simulink model "retro_pid_rootlocus_freq"  (R2021a)
settings: Solver=VariableStepAuto  StartTime=0.0  StopTime=10.0  RelTol=1e-3
values from neighbouring files (symbols this model uses):
  b = 0.1    [controlloPID.m]    (also in modello_CA.m)
  g = 9.8    [controlloPID.m]    (also in modello2.m = 9.81; modello_CA.m = 9.81)
  i = 0.006    [controlloPID.m]    (also in modello_CA.m = 0.00030246)
  Ki = 1    [controlloPID.m]    (also in modello_CA.m = 177.3)
  Kp = 100    [controlloPID.m]    (also in modello_CA.m = 27.59)
  M = 0.5    [controlloPID.m]    (also in modello2.m = 0.04; modello_CA.m = 0.04)
  m = 0.2    [controlloPID.m]    (also in modello2.m = 0.06; modello_CA.m = 0.06)
undefined symbols (not defined in the file or in its folder): k
libraries: pid_lib x1
settings Model: Creator=olegg  LastModifiedBy=olegg

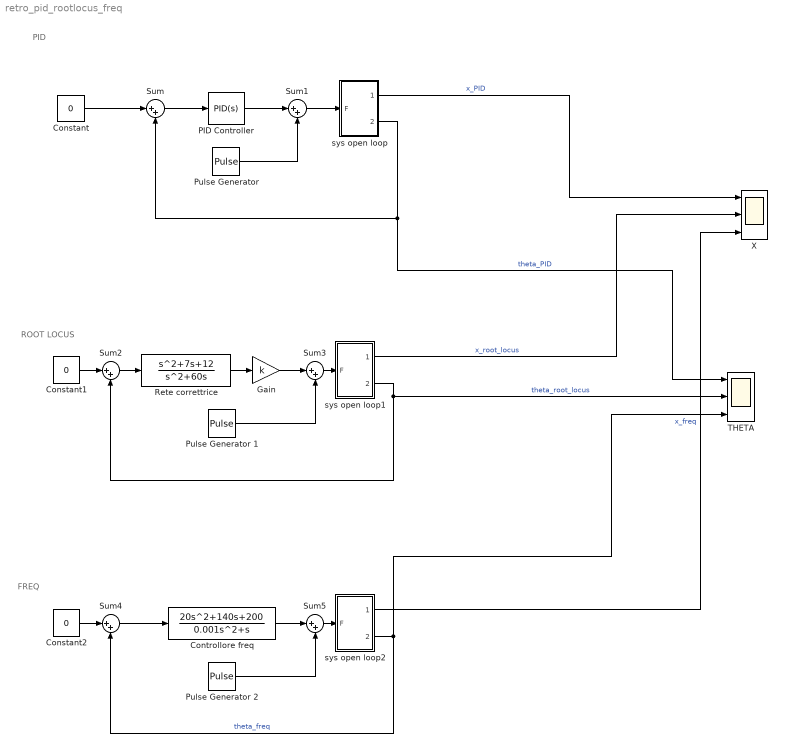
== system retro_pid_rootlocus_freq ==
  note: FREQ
  note: ROOT LOCUS
  note: PID
  Constant : Constant  Value=0
  Constant1 : Constant  Value=0
  Constant2 : Constant  Value=0
  Controllore freq : TransferFcn  Numerator=[20 140 200]  Denominator=[0.001 1 0]
  Gain : Gain  Gain=k
  PID Controller : pid_lib/PID Controller  Controller=PID  Form=Parallel  TimeDomain=Continuous-time  UseExternalTs=off  SampleTime=-1  IntegratorMethod=Forward Euler  FilterMethod=Forward Euler  ControllerParametersSource=internal  P=Kp  I=Ki  D=Kp  UseFilter=on  N=100  TunerSelectOption=Transfer Function Based (PID Tuner App)  InitialConditionSource=internal  InitialConditionForIntegrator=0  InitialConditionForFilter=0  DifferentiatorICPrevScaledInput=0  ExternalReset=none  TrackingMode=off  Kt=1  LimitOutput=off  SatLimitsSource=internal  UpperSaturationLimit=inf  LowerSaturationLimit=-inf  LinearizeAsGain=on  AntiWindupMode=none  Kb=1  POutMin=[]  POutMax=[]  IOutMin=[]  IOutMax=[]  DOutMin=[]  DOutMax=[]  NOutMin=[]  NOutMax=[]  SumOutMin=[]  SumOutMax=[]  SaturationOutMin=[]  SaturationOutMax=[]  PParamMin=[]  PParamMax=[]  IParamMin=[]  IParamMax=[]  DParamMin=[]  DParamMax=[]  NParamMin=[]  NParamMax=[]  KbParamMin=[]  KbParamMax=[]  KtParamMin=[]  KtParamMax=[]  KbOutMin=[]  KbOutMax=[]  KtOutMin=[]  KtOutMax=[]  IntegratorOutMin=[]  IntegratorOutMax=[]  FilterOutMin=[]  FilterOutMax=[]  SumI1OutMin=[]  SumI1OutMax=[]  SumI2OutMin=[]  SumI2OutMax=[]  SumI3OutMin=[]  SumI3OutMax=[]  SumI4OutMin=[]  SumI4OutMax=[]  SumDOutMin=[]  SumDOutMax=[]  DifferentiatorOutMin=[]  DifferentiatorOutMax=[]  FilterDiffOutCoefMin=[]  FilterDiffOutCoefMax=[]  ReciprocalOutMin=[]  ReciprocalOutMax=[]  SumDenOutMin=[]  SumDenOutMax=[]  SumNumOutMin=[]  SumNumOutMax=[]  DivideOutMin=[]  DivideOutMax=[]  UdiffTsProdOutMin=[]  UdiffTsProdOutMax=[]  NTsProdOutMin=[]  NTsProdOutMax=[]  UintegralTsProdOutMin=[]  UintegralTsProdOutMax=[]  UngainTsProdOutMin=[]  UngainTsProdOutMax=[]  IntegratorContinuousStateAttributes=''  IntegratorStateMustResolveToSignalObject=off  IntegratorRTWStateStorageClass=Auto  FilterContinuousStateAttributes=''  FilterStateMustResolveToSignalObject=off  FilterRTWStateStorageClass=Auto  ParallelPVariant=InternalParameters  IdealPVariant=Disabled  IVariant=InternalParameters  DVariant=InternalParameters  IntegratorVariant=Continuous  SatVariant=Disabled  AWVariant=Passthrough  PCopyVariant=Disabled  TRVariant=Disabled  FdbkBlocksVariant=Forward  IdealPFdbkVariant=Disabled  SatFdbkVariant=Disabled  DerivativeFilterVariant=ContFilter  NVariant=InternalParameters  NCopyVariant=Disabled  FilterICVariant=InternalICsFilter  IntegratorICVariant=InternalICs  ExternalResetVariant=Disabled  TRSumVariant=Passthrough  SumFdbkVariant=Disabled  SumVariant=Sum_PID  TsampFilterVariant=InternalTs  TsampNgainVariant=Passthrough  TsampIntegralVariant=Passthrough  ExternalSaturationOutDataTypeStr=Inherit: Same as second input
  "Pulse Generator " : DiscretePulseGenerator  PulseType=Time based  Period=10  PulseWidth=5
  Pulse Generator 1 : DiscretePulseGenerator  PulseType=Time based  Period=10  PulseWidth=5
  Pulse Generator 2 : DiscretePulseGenerator  PulseType=Time based  Period=10  PulseWidth=5
  "Rete correttrice " : TransferFcn  Numerator=[1 7 12]  Denominator=[1 60 0]
  Sum{,1..5} (6 alike) : Sum  Inputs=|++
  THETA : Scope  NumInputPorts=3
  X : Scope  NumInputPorts=3
  sys open loop : Subsystem
  sys open loop1 : Subsystem
  sys open loop2 : Subsystem
  wires:
  Constant/1 -> Sum/1
  Sum/1 -> PID Controller/1
  PID Controller/1 -> Sum1/1
  "Pulse Generator "/1 -> Sum1/2
  Sum1/1 -> sys open loop/1(F)
  sys open loop/2(Out1) -> THETA/1, Sum/2  "theta_PID"
  sys open loop/1(Out2) -> X/1  "x_PID"
  sys open loop1/1(Out2) -> X/2  "x_root_locus"
  "Rete correttrice "/1 -> Gain/1
  Constant1/1 -> Sum2/1
  Sum2/1 -> "Rete correttrice "/1
  Pulse Generator 1/1 -> Sum3/2
  Sum3/1 -> sys open loop1/1(F)
  sys open loop1/2(Out1) -> Sum2/2, THETA/2  "theta_root_locus"
  Gain/1 -> Sum3/1
  Controllore freq/1 -> Sum5/1
  sys open loop2/2(Out1) -> Sum4/2, THETA/3  "theta_freq"
  Constant2/1 -> Sum4/1
  Sum5/1 -> sys open loop2/1(F)
  Pulse Generator 2/1 -> Sum5/2
  sys open loop2/1(Out2) -> X/3  "x_freq"
  Sum4/1 -> Controllore freq/1

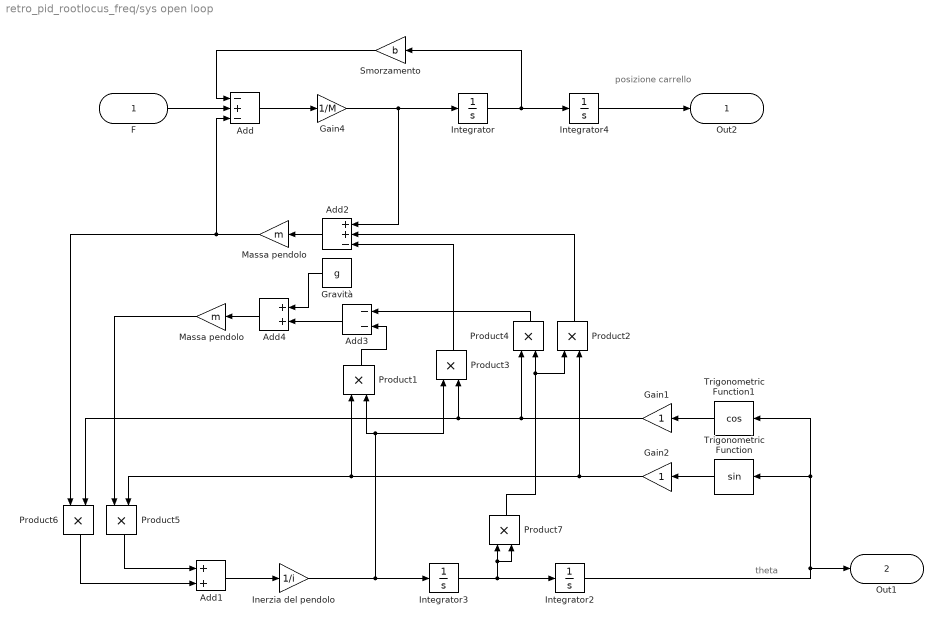
== system retro_pid_rootlocus_freq/sys open loop ==
  note: theta
  note: posizione carrello
  F : Inport
  Add : Sum  Inputs=-+-
  Add1 : Sum
  Add2 : Sum  Inputs=++-
  Add3 : Sum  Inputs=--
  Add4 : Sum
  Gain1 : Gain
  Gain2 : Gain
  Gain4 : Gain  Gain=1/M
  Gravità : Constant  Value=g
  Inerzia del pendolo : Gain  Gain=1/i
  Integrator{,2..4} (4 alike) : Integrator
  Massa pendolo : Gain  Gain=m
  "Massa pendolo " : Gain  Gain=m
  Product{1..7} (7 alike) : Product
  Smorzamento : Gain  Gain=b
  Trigonometric Function : Trigonometry
  Trigonometric Function1 : Trigonometry  Operator=cos
  Out2 : Outport
  Out1 : Outport  Port=2
  wires:
  Integrator2/1 -> Out1/1, Trigonometric Function1/1, Trigonometric Function/1
  F/1 -> Add/2
  Gain4/1 -> Add2/1, Integrator/1
  Add4/1 -> "Massa pendolo "/1
  Inerzia del pendolo/1 -> Integrator3/1, Product3/1, Product1/2
  Smorzamento/1 -> Add/1
  Add3/1 -> Add4/2
  Add2/1 -> Massa pendolo/1
  Gain2/1 -> Product2/2, Product5/2, Product1/1
  Add1/1 -> Inerzia del pendolo/1
  Product4/1 -> Add3/1
  Massa pendolo/1 -> Add/3, Product6/1
  "Massa pendolo "/1 -> Product5/1
  Integrator/1 -> Smorzamento/1, Integrator4/1
  Product2/1 -> Add2/2
  Product1/1 -> Add3/2
  Gravità/1 -> Add4/1
  Product3/1 -> Add2/3
  Integrator3/1 -> Product7/2, Product7/1, Integrator2/1
  Product5/1 -> Add1/1
  Integrator4/1 -> Out2/1
  Add/1 -> Gain4/1
  Gain1/1 -> Product3/2, Product6/2, Product4/1
  Trigonometric Function1/1 -> Gain1/1
  Product7/1 -> Product2/1, Product4/2
  Product6/1 -> Add1/2
  Trigonometric Function/1 -> Gain2/1

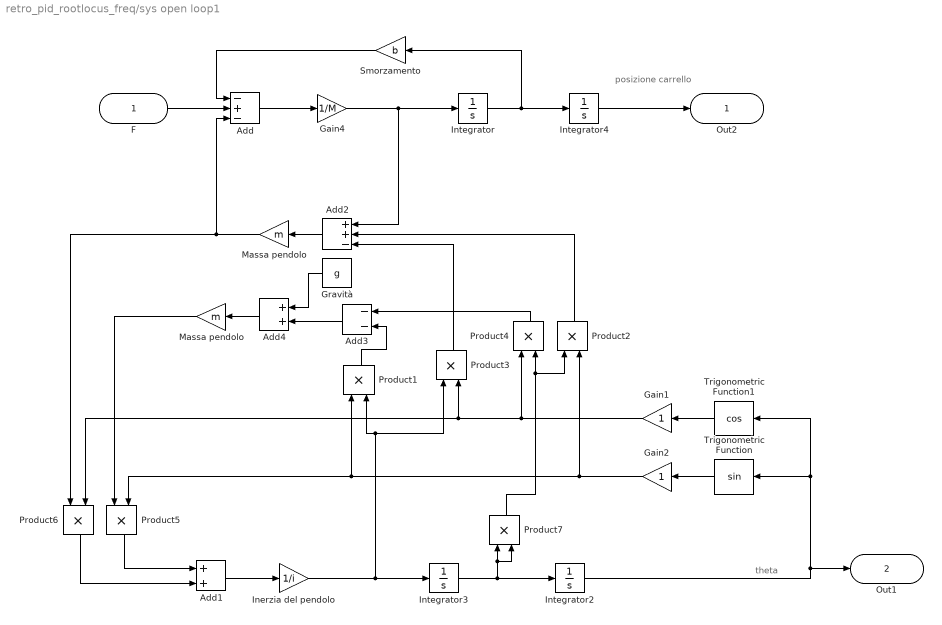
== system retro_pid_rootlocus_freq/sys open loop1 ==
  note: theta
  note: posizione carrello
  F : Inport
  Add : Sum  Inputs=-+-
  Add1 : Sum
  Add2 : Sum  Inputs=++-
  Add3 : Sum  Inputs=--
  Add4 : Sum
  Gain1 : Gain
  Gain2 : Gain
  Gain4 : Gain  Gain=1/M
  Gravità : Constant  Value=g
  Inerzia del pendolo : Gain  Gain=1/i
  Integrator{,2..4} (4 alike) : Integrator
  Massa pendolo : Gain  Gain=m
  "Massa pendolo " : Gain  Gain=m
  Product{1..7} (7 alike) : Product
  Smorzamento : Gain  Gain=b
  Trigonometric Function : Trigonometry
  Trigonometric Function1 : Trigonometry  Operator=cos
  Out2 : Outport
  Out1 : Outport  Port=2
  wires:
  Integrator2/1 -> Out1/1, Trigonometric Function1/1, Trigonometric Function/1
  F/1 -> Add/2
  Gain4/1 -> Add2/1, Integrator/1
  Add4/1 -> "Massa pendolo "/1
  Inerzia del pendolo/1 -> Integrator3/1, Product3/1, Product1/2
  Smorzamento/1 -> Add/1
  Add3/1 -> Add4/2
  Add2/1 -> Massa pendolo/1
  Gain2/1 -> Product2/2, Product5/2, Product1/1
  Add1/1 -> Inerzia del pendolo/1
  Product4/1 -> Add3/1
  Massa pendolo/1 -> Add/3, Product6/1
  "Massa pendolo "/1 -> Product5/1
  Integrator/1 -> Smorzamento/1, Integrator4/1
  Product2/1 -> Add2/2
  Product1/1 -> Add3/2
  Gravità/1 -> Add4/1
  Product3/1 -> Add2/3
  Integrator3/1 -> Product7/2, Product7/1, Integrator2/1
  Product5/1 -> Add1/1
  Integrator4/1 -> Out2/1
  Add/1 -> Gain4/1
  Gain1/1 -> Product3/2, Product6/2, Product4/1
  Trigonometric Function1/1 -> Gain1/1
  Product7/1 -> Product2/1, Product4/2
  Product6/1 -> Add1/2
  Trigonometric Function/1 -> Gain2/1

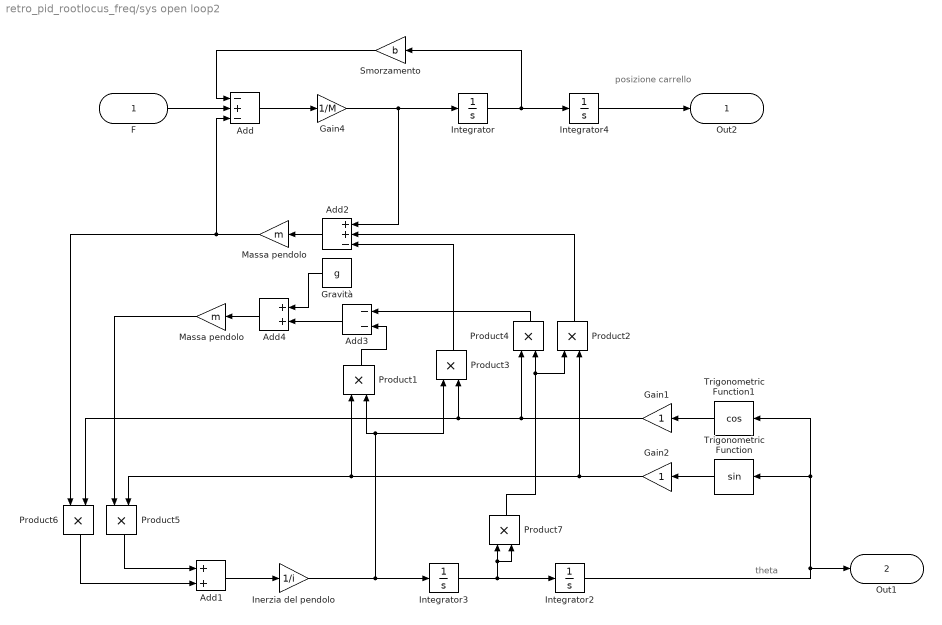
== system retro_pid_rootlocus_freq/sys open loop2 ==
  note: theta
  note: posizione carrello
  F : Inport
  Add : Sum  Inputs=-+-
  Add1 : Sum
  Add2 : Sum  Inputs=++-
  Add3 : Sum  Inputs=--
  Add4 : Sum
  Gain1 : Gain
  Gain2 : Gain
  Gain4 : Gain  Gain=1/M
  Gravità : Constant  Value=g
  Inerzia del pendolo : Gain  Gain=1/i
  Integrator{,2..4} (4 alike) : Integrator
  Massa pendolo : Gain  Gain=m
  "Massa pendolo " : Gain  Gain=m
  Product{1..7} (7 alike) : Product
  Smorzamento : Gain  Gain=b
  Trigonometric Function : Trigonometry
  Trigonometric Function1 : Trigonometry  Operator=cos
  Out2 : Outport
  Out1 : Outport  Port=2
  wires:
  Integrator2/1 -> Out1/1, Trigonometric Function1/1, Trigonometric Function/1
  F/1 -> Add/2
  Gain4/1 -> Add2/1, Integrator/1
  Add4/1 -> "Massa pendolo "/1
  Inerzia del pendolo/1 -> Integrator3/1, Product3/1, Product1/2
  Smorzamento/1 -> Add/1
  Add3/1 -> Add4/2
  Add2/1 -> Massa pendolo/1
  Gain2/1 -> Product2/2, Product5/2, Product1/1
  Add1/1 -> Inerzia del pendolo/1
  Product4/1 -> Add3/1
  Massa pendolo/1 -> Add/3, Product6/1
  "Massa pendolo "/1 -> Product5/1
  Integrator/1 -> Smorzamento/1, Integrator4/1
  Product2/1 -> Add2/2
  Product1/1 -> Add3/2
  Gravità/1 -> Add4/1
  Product3/1 -> Add2/3
  Integrator3/1 -> Product7/2, Product7/1, Integrator2/1
  Product5/1 -> Add1/1
  Integrator4/1 -> Out2/1
  Add/1 -> Gain4/1
  Gain1/1 -> Product3/2, Product6/2, Product4/1
  Trigonometric Function1/1 -> Gain1/1
  Product7/1 -> Product2/1, Product4/2
  Product6/1 -> Add1/2
  Trigonometric Function/1 -> Gain2/1
